simulink model "T6_12"  (R2021a)
settings: Solver=VariableStepAuto  StartTime=0.0  StopTime=2.0  RelTol=1e-3
values from neighbouring files (symbols this model uses):
  A = [2 6; 1 0]    [myCode.m]
  B = [4;1]    [myCode.m]
  Bf = [1;3]    [myCode.m]
  C = [2 0]    [myCode.m]
  D = 6    [myCode.m]
  Hg = H_g    [myCode.m]
  Ke = K_(1), Kx = [K_(2) K_(3)]    [myCode.m]
undefined symbols (not defined in the file or in its folder): Kx, T2
settings Model: Creator=fedor  LastModifiedBy=fedor

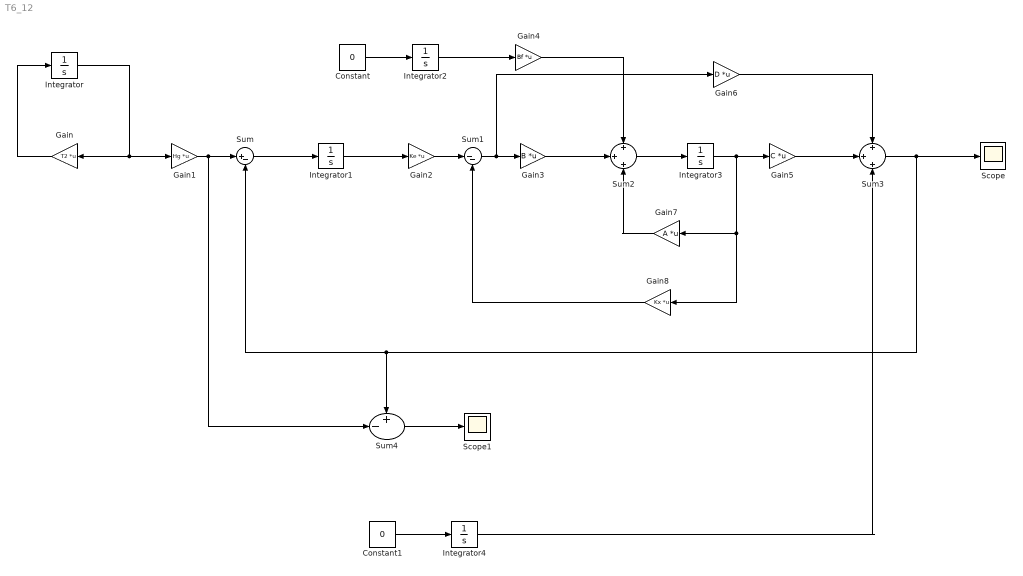
== system T6_12 ==
  Constant : Constant  Value=0
  Constant1 : Constant  Value=0
  Gain : Gain  Gain=T2  Multiplication=Matrix(K*u)
  Gain1 : Gain  Gain=Hg  Multiplication=Matrix(K*u)
  Gain2 : Gain  Gain=Ke  Multiplication=Matrix(K*u)
  Gain3 : Gain  Gain=B  Multiplication=Matrix(K*u)
  Gain4 : Gain  Gain=Bf  Multiplication=Matrix(K*u)
  Gain5 : Gain  Gain=C  Multiplication=Matrix(K*u)
  Gain6 : Gain  Gain=D  Multiplication=Matrix(K*u)
  Gain7 : Gain  Gain=A  Multiplication=Matrix(K*u)
  Gain8 : Gain  Gain=Kx  Multiplication=Matrix(K*u)
  Integrator : Integrator  InitialCondition=1
  Integrator1 : Integrator
  Integrator2 : Integrator  InitialCondition=1
  Integrator3 : Integrator
  Integrator4 : Integrator  InitialCondition=1
  Scope : Scope
  Scope1 : Scope
  Sum : Sum  Inputs=|+-
  Sum1 : Sum  Inputs=|--
  Sum2 : Sum  Inputs=+|+|+
  Sum3 : Sum  Inputs=+|+|+
  Sum4 : Sum  Inputs=+-|
  wires:
  Gain/1 -> Integrator/1
  Integrator/1 -> Gain1/1, Gain/1
  Gain1/1 -> Sum4/2, Sum/1
  Sum/1 -> Integrator1/1
  Integrator1/1 -> Gain2/1
  Gain2/1 -> Sum1/1
  Sum1/1 -> Gain6/1, Gain3/1
  Gain3/1 -> Sum2/2
  Gain4/1 -> Sum2/1
  Integrator2/1 -> Gain4/1
  Constant/1 -> Integrator2/1
  Sum2/1 -> Integrator3/1
  Integrator3/1 -> Gain8/1, Gain7/1, Gain5/1
  Gain5/1 -> Sum3/2
  Gain6/1 -> Sum3/1
  Sum3/1 -> Sum4/1, Sum/2, Scope/1
  Gain7/1 -> Sum2/3
  Gain8/1 -> Sum1/2
  Sum4/1 -> Scope1/1
  Integrator4/1 -> Sum3/3
  Constant1/1 -> Integrator4/1
